simulink model "senal_vel_trapezoidal"  (R2023b)
settings: Solver=VariableStepAuto  StartTime=0.0  StopTime=15  RelTol=1e-3
libraries: simulink x8
settings Model: Creator=rodri  LastModifiedBy=rodri

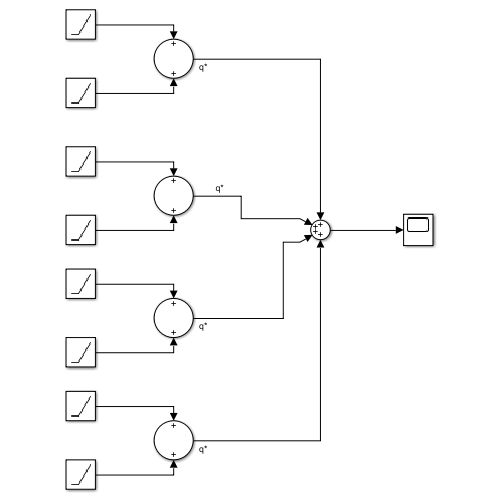
[thumbnail: Simulink's stored preview of the top-level diagram]
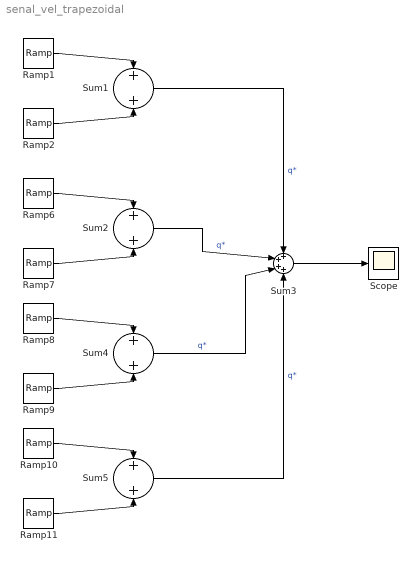
== system senal_vel_trapezoidal ==
  Ramp1 : simulink/Sources/Ramp  slope=150.8/0.2  start=0  InitialOutput=0
  Ramp10 : simulink/Sources/Ramp  slope=150.8/0.2  start=14.8  InitialOutput=0
  Ramp11 : simulink/Sources/Ramp  slope=-150.8/0.2  start=15  InitialOutput=0
  Ramp2 : simulink/Sources/Ramp  slope=-150.8/0.2  start=0.2  InitialOutput=0
  Ramp6 : simulink/Sources/Ramp  slope=-150.8/0.2  start=4.8  InitialOutput=0
  Ramp7 : simulink/Sources/Ramp  slope=150.8/0.2  start=5  InitialOutput=0
  Ramp8 : simulink/Sources/Ramp  slope=-150.8/0.2  start=10  InitialOutput=0
  Ramp9 : simulink/Sources/Ramp  slope=150.8/0.2  start=10.2  InitialOutput=0
  Scope : Scope
  Sum{1..2,4..5} (4 alike) : Sum
  Sum3 : Sum  Inputs=++++
  wires:
  Sum4/1 -> Sum3/3  "q*"
  Sum1/1 -> Sum3/1  "q*"
  Sum3/1 -> Scope/1
  Ramp10/1 -> Sum5/1
  Ramp11/1 -> Sum5/2
  Sum5/1 -> Sum3/4  "q*"
  Ramp9/1 -> Sum4/2
  Ramp2/1 -> Sum1/2
  Ramp1/1 -> Sum1/1
  Ramp8/1 -> Sum4/1
  Sum2/1 -> Sum3/2  "q*"
  Ramp6/1 -> Sum2/1
  Ramp7/1 -> Sum2/2
